simulink model "simulation"  (R2026a)
settings: Solver=VariableStepAuto
InitFcn:
  | setup
values from neighbouring files (symbols this model uses):
  r = sqrt(ms)    [run_monte_carlo.m]
undefined symbols (not defined in the file or in its folder): F, Light, MIL, params
libraries: aerolibadyn x1, aerolibwind2 x1, uavutilslib x1
settings Model: Creator=chris  LastModifiedBy=maxim

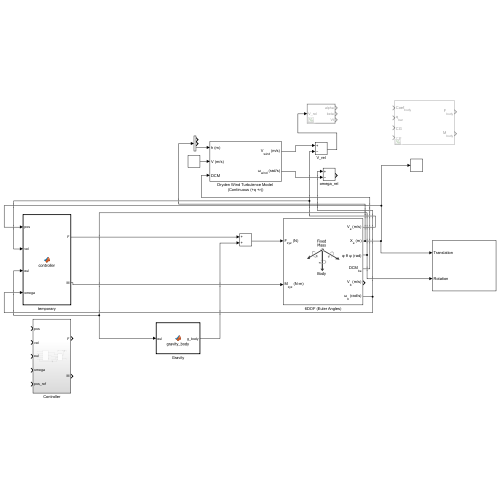
[thumbnail: Simulink's stored preview of the top-level diagram]
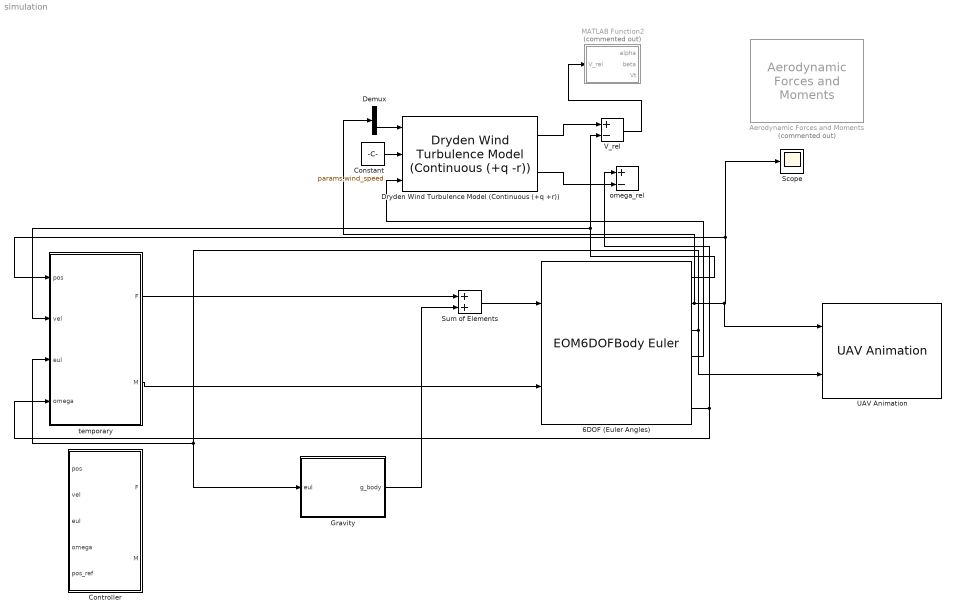
== system simulation ==
  6DOF (Euler Angles) : EOM6DOFBodyEuler
  "Aerodynamic Forces and Moments " : aerolibadyn/Aerodynamic Forces and Moments   Commented=on  inputAxes=Body  outputForceAxes=Body  outputMomentAxes=Body  S=1  b=1  cbar=1
  Constant : Constant  Value=params.wind_speed
      settings: OpenFcn=setup
  Controller : Subsystem
  Demux : Demux  Outputs=3
  Dryden Wind Turbulence Model (Continuous (+q +r)) : aerolibwind2/Dryden Wind Turbulence Model  (Continuous (+q -r))  units=Metric (MKS)  spec=MIL-F-8785C  model=Continuous Dryden (+q +r)  W20=15  Wdeg=0  TurbProb=10^-2 - Light  L_high=533.4  Wingspan=10  ts=0.1  Seed=[23341 23342 23343 23344]  T_on=on
      settings: LibrarySourceBlock=|
      | aerolibwind2/Dryden Wind Turbulence Model
      | (Continuous (+q +r))
  Gravity : MATLAB Function  TreatAsAtomicUnit=on
  MATLAB Function2 : MATLAB Function  Commented=on  TreatAsAtomicUnit=on
  Scope : Scope
      settings: ActiveDisplayYMinimum=-31.992799927432571  ActiveDisplayYMaximum=305.00152772715626
  Sum of Elements : Sum
  UAV Animation : uavutilslib/UAV Animation  NumUAV=1  DynamicUAVConfig=off  UAVType=Multirotor  UAVSize=10  UAVColor=[1 0 0]  UAVTrajectoryAlpha=1  AlwaysShowAnimation=on  AxisLimits=[-100 100;-100 100;-100 100]  TrajectoryBufferSize=100000  InertialZDirection=Down  RotationFormat=Euler ZYX  DrawMarkers=off  SampleTime=0.05
  V_rel : Sum  Inputs=+-
  omega_rel : Sum  Inputs=+-
  temporary : MATLAB Function  TreatAsAtomicUnit=on
  wires:
  temporary/2(M) -> 6DOF (Euler Angles)/2
  6DOF (Euler Angles)/6 -> omega_rel/1, temporary/4(omega)
  6DOF (Euler Angles)/2 -> Demux/1, UAV Animation/1, Scope/1, temporary/1(pos)
  6DOF (Euler Angles)/1 -> V_rel/2, temporary/2(vel)
  6DOF (Euler Angles)/3 -> UAV Animation/2, Gravity/1(eul), temporary/3(eul)
  Constant/1 -> Dryden Wind Turbulence Model (Continuous (+q +r))/2
  6DOF (Euler Angles)/4 -> Dryden Wind Turbulence Model (Continuous (+q +r))/3
  Demux/3 -> Dryden Wind Turbulence Model (Continuous (+q +r))/1
  temporary/1(F) -> Sum of Elements/1
  Gravity/1(g_body) -> Sum of Elements/2
  Sum of Elements/1 -> 6DOF (Euler Angles)/1
  Dryden Wind Turbulence Model (Continuous (+q +r))/1 -> V_rel/1
  Dryden Wind Turbulence Model (Continuous (+q +r))/2 -> omega_rel/2
  V_rel/1 -> MATLAB Function2/1(V_rel)

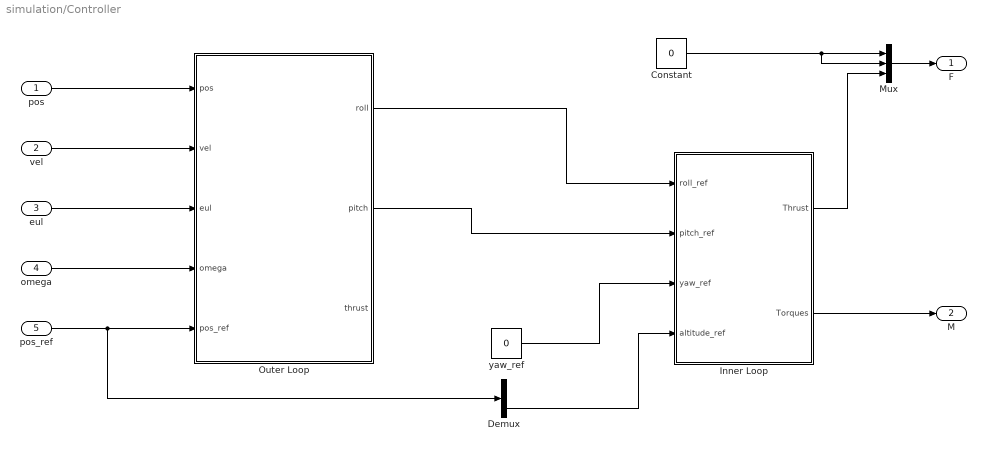
== system simulation/Controller ==
  pos : Inport
  vel : Inport  Port=2
  eul : Inport  Port=3
  omega : Inport  Port=4
  pos_ref : Inport  Port=5
  Constant : Constant  Value=0
  Demux : Demux  Outputs=3
  Inner Loop : Subsystem
  Mux : Mux  Inputs=3
  Outer Loop : Subsystem
  yaw_ref : Constant  Value=0
  F : Outport
  M : Outport  Port=2
  wires:
  pos/1 -> Outer Loop/1(pos)
  vel/1 -> Outer Loop/2(vel)
  pos_ref/1 -> Outer Loop/5(pos_ref), Demux/1
  eul/1 -> Outer Loop/3(eul)
  Inner Loop/2(Torques) -> M/1
  Inner Loop/1(Thrust) -> Mux/3
  Constant/1 -> Mux/1, Mux/2
  Mux/1 -> F/1
  Outer Loop/1(roll) -> Inner Loop/1(roll_ref)
  yaw_ref/1 -> Inner Loop/3(yaw_ref)
  Demux/3 -> Inner Loop/4(altitude_ref)
  omega/1 -> Outer Loop/4(omega)
  Outer Loop/2(pitch) -> Inner Loop/2(pitch_ref)

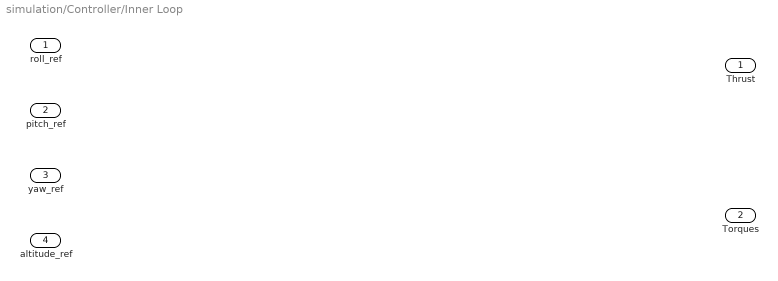
== system simulation/Controller/Inner Loop ==
  roll_ref : Inport
  pitch_ref : Inport  Port=2
  yaw_ref : Inport  Port=3
  altitude_ref : Inport  Port=4
  Thrust : Outport
  Torques : Outport  Port=2

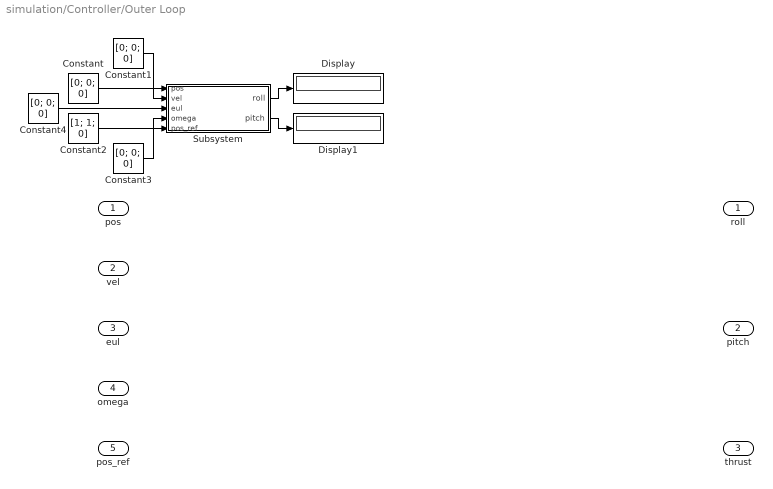
== system simulation/Controller/Outer Loop ==
  pos : Inport
  vel : Inport  Port=2
  eul : Inport  Port=3
  omega : Inport  Port=4
  pos_ref : Inport  Port=5
  Constant{,1,3..4} (4 alike) : Constant  Value=[0; 0; 0]
  Constant2 : Constant  Value=[1; 1; 0]
  Display : Display
  Display1 : Display
  Subsystem : Subsystem
  roll : Outport
  pitch : Outport  Port=2
  thrust : Outport  Port=3
  wires:
  Subsystem/2(pitch) -> Display1/1
  Constant1/1 -> Subsystem/2(vel)
  Constant4/1 -> Subsystem/3(eul)
  Subsystem/1(roll) -> Display/1
  Constant3/1 -> Subsystem/4(omega)
  Constant2/1 -> Subsystem/5(pos_ref)
  Constant/1 -> Subsystem/1(pos)

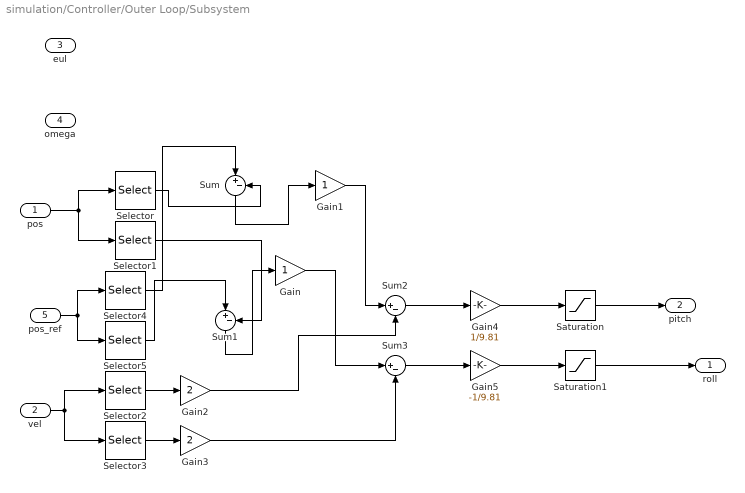
== system simulation/Controller/Outer Loop/Subsystem ==
  pos : Inport
  vel : Inport  Port=2
  eul : Inport  Port=3
  omega : Inport  Port=4
  pos_ref : Inport  Port=5
  Gain : Gain
  Gain1 : Gain
  Gain2 : Gain  Gain=2
  Gain3 : Gain  Gain=2
  Gain4 : Gain  Gain=1/9.81
  Gain5 : Gain  Gain=-1/9.81
  Saturation : Saturate
  Saturation1 : Saturate
  Selector : Selector  InputPortWidth=3  IndexOptions=Index vector (dialog)  Indices=1  OutputSizes=1
  Selector1 : Selector  InputPortWidth=3  IndexOptions=Index vector (dialog)  Indices=2  OutputSizes=1
  Selector2 : Selector  InputPortWidth=3  IndexOptions=Index vector (dialog)  Indices=1  OutputSizes=1
  Selector3 : Selector  InputPortWidth=3  IndexOptions=Index vector (dialog)  Indices=2  OutputSizes=1
  Selector4 : Selector  InputPortWidth=3  IndexOptions=Index vector (dialog)  Indices=1  OutputSizes=1
  Selector5 : Selector  InputPortWidth=3  IndexOptions=Index vector (dialog)  Indices=2  OutputSizes=1
  Sum{,1..3} (4 alike) : Sum  Inputs=|+-
  roll : Outport
  pitch : Outport  Port=2
  wires:
  Gain4/1 -> Saturation/1
  Selector2/1 -> Gain2/1
  Sum1/1 -> Gain/1
  pos/1 -> Selector1/1, Selector/1
  pos_ref/1 -> Selector5/1, Selector4/1
  Gain/1 -> Sum3/1
  Gain5/1 -> Saturation1/1
  Gain1/1 -> Sum2/1
  Selector1/1 -> Sum1/2
  Sum3/1 -> Gain5/1
  Sum/1 -> Gain1/1
  Selector5/1 -> Sum1/1
  Selector/1 -> Sum/2
  Gain3/1 -> Sum3/2
  Sum2/1 -> Gain4/1
  vel/1 -> Selector2/1, Selector3/1
  Selector3/1 -> Gain3/1
  Gain2/1 -> Sum2/2
  Selector4/1 -> Sum/1
  Saturation1/1 -> roll/1
  Saturation/1 -> pitch/1

== matlab function simulation/Gravity ==
  data: eul input; g_body output; params parameter
function g_body = gravity_body(eul, params)
% eul = [roll pitch yaw] from the 6DOF block (rad). NED: +z down.
    g_world = [0; 0; params.m * params.g];
    R = eul2rotm([eul(3) eul(2) eul(1)]);   % eul2rotm wants [yaw pitch roll]
    g_body = R' * g_world;                   % world->body
end

== matlab function simulation/temporary ==
  data: pos input; F output; vel input; eul input; omega input; M output
function [F, M] = controller(pos, vel, eul, omega)
    F = [0; 0; -10];   % thrust in body/world z, per block's frame convention
    M = [1; 1; 1];
end

== matlab function simulation/MATLAB Function2 ==
  data: V_rel input; alpha output; beta output; Vt output
function [alpha,beta,Vt] = airdata_calc(V_rel)
    u = V_rel(1);
    v = V_rel(2);
    w = V_rel(3);

    Vt = sqrt(u^2 + v^2 + w^2);
    if Vt < 1e-6
        alpha = 0;
        beta = 0;
   
    else
        alpha = atan(w,u);
        beta = asin(v/Vt);
    end
end
